simulink model "Model_3"  (R2020b)
settings: Solver=VariableStepAuto  StartTime=0.0  StopTime=10.0  RelTol=1e-3
settings Model: Creator=Akarsh  LastModifiedBy=Akarsh

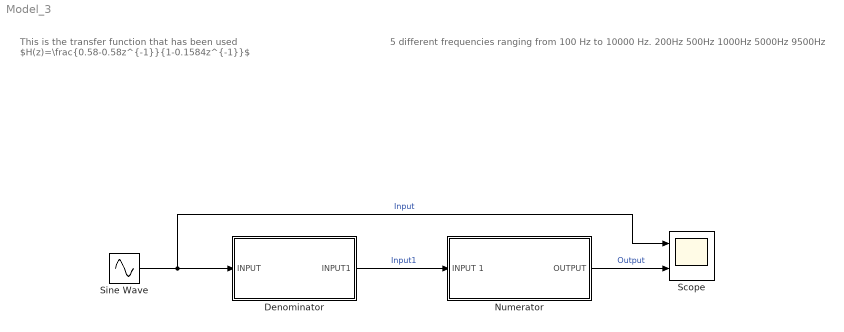
== system Model_3 ==
  note: This is the transfer function that has been used
      | $H(z)=\frac{0.58-0.58z^{-1}}{1-0.1584z^{-1}}$
  note: 5 different frequencies ranging from 100 Hz to 10000 Hz.
      | 200Hz
      | 500Hz
      | 1000Hz
      | 5000Hz
      | 9500Hz
  Denominator : Subsystem  TreatAsAtomicUnit=on
  Numerator : Subsystem  TreatAsAtomicUnit=on
  Scope : Scope  NumInputPorts=2
  Sine Wave : Sin  Frequency=2*pi*1000  SampleTime=0
  wires:
  Denominator/1(INPUT1) -> Numerator/1(INPUT 1)  "Input1"
  Numerator/1(OUTPUT) -> Scope/2  "Output"
  Sine Wave/1 -> Scope/1, Denominator/1(INPUT)  "Input"

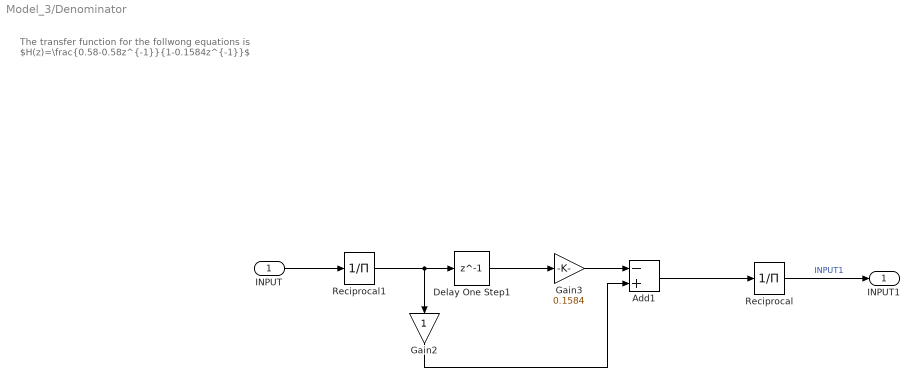
== system Model_3/Denominator ==
  note: The transfer function for the follwong equations is
      | $H(z)=\frac{0.58-0.58z^{-1}}{1-0.1584z^{-1}}$
  INPUT : Inport
  Add1 : Sum  Inputs=-+
  Delay One Step1 : Delay  DelayLength=1
  Gain2 : Gain
  Gain3 : Gain  Gain=0.1584
  Reciprocal : Product  Inputs=/
  Reciprocal1 : Product  Inputs=/
  INPUT1 : Outport
  wires:
  Add1/1 -> Reciprocal/1
  Reciprocal/1 -> INPUT1/1  "INPUT1"
  Delay One Step1/1 -> Gain3/1
  Reciprocal1/1 -> Delay One Step1/1, Gain2/1
  Gain2/1 -> Add1/2
  Gain3/1 -> Add1/1
  INPUT/1 -> Reciprocal1/1

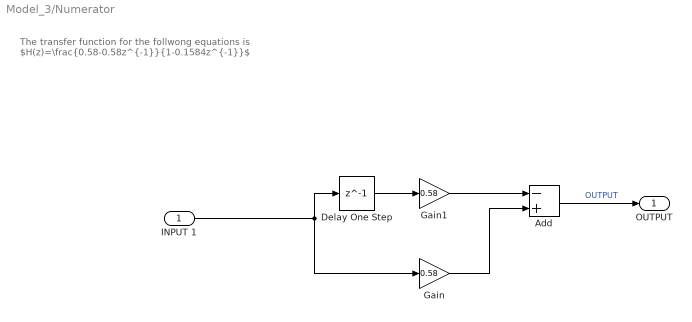
== system Model_3/Numerator ==
  note: The transfer function for the follwong equations is
      | $H(z)=\frac{0.58-0.58z^{-1}}{1-0.1584z^{-1}}$
  INPUT 1 : Inport
  Add : Sum  Inputs=-+
  Delay One Step : Delay  DelayLength=1
  Gain : Gain  Gain=0.58
  Gain1 : Gain  Gain=0.58
  OUTPUT : Outport
  wires:
  Gain1/1 -> Add/1
  Gain/1 -> Add/2
  INPUT 1/1 -> Delay One Step/1, Gain/1
  Delay One Step/1 -> Gain1/1
  Add/1 -> OUTPUT/1  "OUTPUT"
